simulink model "dual_magnet_model"  (R2016a)
settings: Solver=VariableStepAuto  StartTime=0.0  StopTime=.01  RelTol=1e-3
undefined symbols (not defined in the file): K
settings Model: Creator=manuel  LastModifiedBy=manuel

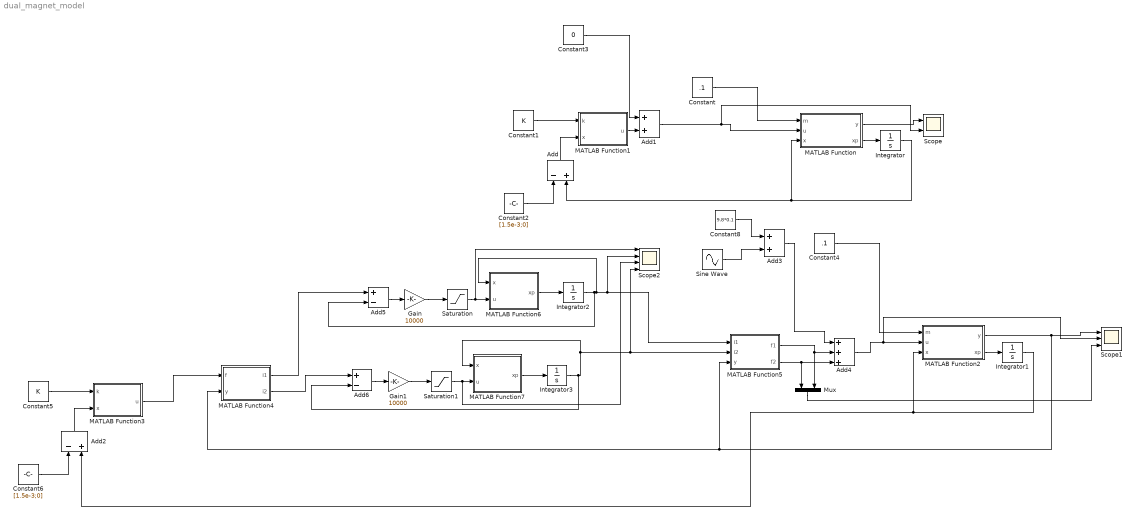
== system dual_magnet_model ==
  Add : Sum  Inputs=-+
  Add1 : Sum
  Add2 : Sum  Inputs=-+
  Add3 : Sum
  Add4 : Sum  Inputs=+++
  Add5 : Sum  Inputs=+-
  Add6 : Sum  Inputs=+-
  Constant : Constant  Value=.1
  Constant1 : Constant  Value=K
  Constant2 : Constant  Value=[1.5e-3;0]
  Constant3 : Constant  Value=0
  Constant4 : Constant  Value=.1
  Constant5 : Constant  Value=K
  Constant6 : Constant  Value=[1.5e-3;0]
  Constant8 : Constant  Value=9.8*0.1
  Gain : Gain  Gain=10000
  Gain1 : Gain  Gain=10000
  Integrator : Integrator  InitialCondition=[1.6e-3;0]  LimitOutput=on  UpperSaturationLimit=[2e-3;inf]  LowerSaturationLimit=[1e-3;-inf]
  Integrator1 : Integrator  InitialCondition=[1.6e-3;0]  LimitOutput=on  UpperSaturationLimit=[2e-3;inf]  LowerSaturationLimit=[1e-3;-inf]
  Integrator2 : Integrator  InitialCondition=[0]  UpperSaturationLimit=[inf]  LowerSaturationLimit=[-inf]
  Integrator3 : Integrator  InitialCondition=[0]  UpperSaturationLimit=[inf]  LowerSaturationLimit=[-inf]
  MATLAB Function : MATLAB Function  TreatAsAtomicUnit=on
  MATLAB Function1 : MATLAB Function  TreatAsAtomicUnit=on
  MATLAB Function2 : MATLAB Function  TreatAsAtomicUnit=on
  MATLAB Function3 : MATLAB Function  TreatAsAtomicUnit=on
  MATLAB Function4 : MATLAB Function  TreatAsAtomicUnit=on
  MATLAB Function5 : MATLAB Function  TreatAsAtomicUnit=on
  MATLAB Function6 : MATLAB Function  TreatAsAtomicUnit=on
  MATLAB Function7 : MATLAB Function  TreatAsAtomicUnit=on
  Mux : Mux  Inputs=2
  Saturation : Saturate  UpperLimit=24  LowerLimit=-24
  Saturation1 : Saturate  UpperLimit=24  LowerLimit=-24
  Scope : Scope  NumInputPorts=2
  Scope1 : Scope  NumInputPorts=3
  Scope2 : Scope  NumInputPorts=4
  Sine Wave : Sin  Amplitude=2  Frequency=2*pi*100  SampleTime=0
  wires:
  MATLAB Function/2(xp) -> Integrator/1
  Integrator/1 -> MATLAB Function/3(x), Add/2
  Constant/1 -> MATLAB Function/1(m)
  MATLAB Function/1(y) -> Scope/1
  Constant1/1 -> MATLAB Function1/1(k)
  Constant2/1 -> Add/1
  Add/1 -> MATLAB Function1/2(x)
  MATLAB Function1/1(u) -> Add1/2
  Constant3/1 -> Add1/1
  Add1/1 -> Scope/2, MATLAB Function/2(u)
  MATLAB Function2/2(xp) -> Integrator1/1
  Integrator1/1 -> Add2/2, MATLAB Function2/3(x)
  Constant4/1 -> MATLAB Function2/1(m)
  MATLAB Function2/1(y) -> Scope1/1, MATLAB Function5/3(y), MATLAB Function4/2(y)
  Constant5/1 -> MATLAB Function3/1(k)
  Constant6/1 -> Add2/1
  Add2/1 -> MATLAB Function3/2(x)
  MATLAB Function5/2(f2) -> Add4/3, Mux/1
  Add4/1 -> Scope1/2, MATLAB Function2/2(u)
  MATLAB Function5/1(f1) -> Add4/2, Mux/2
  Mux/1 -> Scope1/3
  MATLAB Function6/1(xp) -> Integrator2/1
  Saturation/1 -> Scope2/1, MATLAB Function6/2(u)
  Integrator2/1 -> Add5/2, MATLAB Function6/1(x), Scope2/2, MATLAB Function5/1(i1)
  Add5/1 -> Gain/1
  Gain/1 -> Saturation/1
  MATLAB Function7/1(xp) -> Integrator3/1
  Saturation1/1 -> Scope2/3, MATLAB Function7/2(u)
  Integrator3/1 -> Scope2/4, MATLAB Function5/2(i2), MATLAB Function7/1(x), Add6/2
  Add6/1 -> Gain1/1
  Gain1/1 -> Saturation1/1
  MATLAB Function4/1(i1) -> Add5/1
  MATLAB Function4/2(i2) -> Add6/1
  MATLAB Function3/1(u) -> MATLAB Function4/1(f)
  Add3/1 -> Add4/1
  Constant8/1 -> Add3/1
  Sine Wave/1 -> Add3/2

== matlab function dual_magnet_model/MATLAB Function1 ==
  data: k input; x input; u output
function u = fcn(k,x)
%#codegen

u = -k'*x;

== matlab function dual_magnet_model/MATLAB Function ==
  data: m input; u input; x input; y output; xp output
function [y,xp] = mass_model(m,u,x)
%#codegen
A = [0 1
     0 0];
B = [0;
     1/m];
C = [1 0];

xp = A*x + B*u;
y = C*x;

== matlab function dual_magnet_model/MATLAB Function2 ==
  data: m input; u input; x input; y output; xp output
function [y,xp] = mass_model(m,u,x)
%#codegen
A = [0 1
     0 0];
B = [0;
     1/m];
C = [1 0];

xp = A*x + B*u;
y = C*x;

== matlab function dual_magnet_model/MATLAB Function3 ==
  data: k input; x input; u output
function u = fcn(k,x)
%#codegen

u = -k'*x;

== matlab function dual_magnet_model/MATLAB Function4 ==
  data: f input; i1 output; i2 output; y input
function [i1,i2] = fcn(f,y)
%#codegen

k = 9.8*(2e-3)^2;

y2 = 3.0e-3 - y;
y1 = y;

use_electromagnet_1 = f < 0;
use_electromagnet_2 = f > 0;
if(use_electromagnet_1)
i1 = sqrt(y1^2*(-f)*(1/k));
else
i1 = 0;
end

if(use_electromagnet_2)
i2 = sqrt(y2^2*f*(1/k));
else
i2 = 0;
end

== matlab function dual_magnet_model/MATLAB Function5 ==
  data: i1 input; f1 output; i2 input; y input; f2 output
function [f1,f2]  = fcn(i1,i2,y)
%#codegen

k = 9.8*(2e-3)^2;

y1 = y;
y2 = 3.0e-3 - y;

f1 = -k*(i1/y1)^2;
f2 = k*(i2/y2)^2;

== matlab function dual_magnet_model/MATLAB Function6 ==
  data: x input; xp output; u input
function xp  = electrical_model(x,u)

L = 0.010;
R = 0.25;

A = [-R/L];
B = [1/L];
xp = A*x + B*u;

== matlab function dual_magnet_model/MATLAB Function7 ==
  data: x input; xp output; u input
function xp  = electrical_model(x,u)

L = 0.010;
R = 0.25;

A = [-R/L];
B = [1/L];
xp = A*x + B*u;
